simulink library "SUB_ECU_L4_MABX_HW_Interface_PIC_KW"  (R2018a)
settings: Solver=VariableStepAuto  StartTime=0.0  StopTime=10.0  RelTol=1e-3
PostLoadFcn:
  | , if any(exist('dsrtsu_mdlpostloadfcn', 'file') == [2, 3, 6]), try dsrtsu_mdlpostloadfcn('Execute', bdroot); catch fprintf('Error in PostLoadFcn (dsrtsu_mdlpostloadfcn) for model "%s":\n %s\n', bdroot, lasterr); end, end,
undefined symbols (not defined in the file or in its folder): CANR_PROPB_REAX_3_13_CHANNEL_APV, CANR_PROPB_REAX_4_13_CHANNEL_APV, CANR_PROPB_XPR_1_50_CHANNEL_APV, ENUM_CAN_RX_T, ENUM_CAN_TX_T, ENUM_REAX_OPERATION_MODE_T, ENUM_SIGNAL_HEALTH_T, ENUM_XBR_CONTROL_MODE_T, ENUM_XBR_EBI_MODE_T, ENUM_XBR_PASS_THROUGH_ACTIVE_T, ENUM_XBR_PRIORITY_T, ENUM_XPR_INHIBIT_PARK_MANUAL_T, ENUM_XPR_INHIBIT_UNPARK_MANUAL_T, ENUM_XPR_PARK_MANUAL_T, ENUM_XPR_UNPARK_MANUAL_T, PROPB_REAX_1_E4_DES_POS_SIG_SRC_APV, PROPB_REAX_1_E4_DESIRED_OPMODE_APV, PROPB_REAX_1_E4_DESIRED_POSITION_APV, PROPB_REAX_CHANNEL_APV, ptc_matlab_lib
libraries: PTC_MBDS_LIB x292, rtican x158, simulink x58, EmE_MBD_Blockset x38, rti1401lib_dio_type4 x13, simulink_need_slupdate x7, rti1401lib_adc_type4 x3, rtmapslib x3, $bdroot x3, dsa_tcpip_lib x2, SUB_ECU_L4_MABX_HW_Interface_PTC_1571 x1, rtitasklib x1
(part 7 of 48)

== system SUB_ECU_L4_MABX_HW_Interface_PIC_KW/CAN_Out_PIC_KW/CAN_TX_20ms/Encode_PropB_XBR_B3 ==
  note: This might cause a limit cycle, why switch pass through mode based on braking error
  In : Inport
  Bus Creator1 : BusCreator  Inputs=7
  Bus Creator2 : BusCreator  Inputs=7
  Bus Selector2 : BusSelector  OutputSignals=10msTask.BrakeCtrl.BrakingPID_Y,10msTask.BrakeCtrl.BrakingControlActive,INPUTS.DIO_Bus.OperatorEnableSwitch
  Constant10 : Constant  Value=ENUM_XBR_PASS_THROUGH_ACTIVE_T.NOT_ACTIVE
  Constant2 : Constant  Value=-15.687
  Constant4 : Constant  Value=0
  Constant7 : Constant  Value=ENUM_XBR_PASS_THROUGH_ACTIVE_T.ACTIVE
  Constant8 : Constant  Value=ENUM_XBR_PASS_THROUGH_ACTIVE_T.ERROR
  Constant9 : Constant  Value=ENUM_XBR_PASS_THROUGH_ACTIVE_T.NOT_AVAILABLE
  DECEL_GOV_XBR_URGENCY_MPV : Lookup_n-D  NumberOfTableDimensions=1  BreakpointsForDimension1=[-15.687 -2 -1.5 -1.2 -1.1 -1 -0.9 0]  Table=[100 50 20 15 15 15 10 10]  ExtrapMethod=Clip  UseLastTableValue=on  InputSameDT=on
      settings: AttributesFormatString=|
      | X: %<BreakpointsForDimension1>
      | Y: %<Table>
  Divide1 : Product  Inputs=**  InputSameDT=on
  If_Then_Else : EmE_MBD_Blockset/Signal Routing/If_Then_Else
      settings: SourceProductName=PACCAR EmE MBD Blockset
  Multiport Switch : MultiPortSwitch  DataPortOrder=Zero-based contiguous  Inputs=4  DiagnosticForDefault=None  zeroidx=on  InputSameDT=on
  Switch1 : Switch  Criteria=u2 ~= 0
  Terminator1 : Terminator
  XBRControlMode : Constant  Value=ENUM_XBR_CONTROL_MODE_T.ACCEL_CTRL_WITH_MAX_MODE
  XBRControlModeOVR : Constant  Value=ENUM_XBR_CONTROL_MODE_T.ACCEL_CTRL_WITH_MAX_MODE
  XBREnduranceBrakeIntegrationMode : Constant  Value=ENUM_XBR_EBI_MODE_T.EBI_ALLOWED
  XBREnduranceBrakeIntegrationModeOVR : Constant  Value=ENUM_XBR_EBI_MODE_T.EBI_ALLOWED
  XBRExternalAccelDemandOVR : Constant  Value=0
  XBRPassThroughActiveOVR : Constant  Value=ENUM_XBR_PASS_THROUGH_ACTIVE_T.ACTIVE
  XBRPassThroughEnabled : Constant
  XBRPassThroughEnabledOVR : Constant
  XBRPriority : Constant  Value=ENUM_XBR_PRIORITY_T.MEDIUM_PRIORITY
  XBRPriorityOVR : Constant  Value=ENUM_XBR_PRIORITY_T.MEDIUM_PRIORITY
  XBRUrgency : Constant  Value=25
  XBRUrgencyOVR : Constant  Value=25
  XBRValueOverride : Constant  Value=false
  Out : Outport
  wires:
  Constant4/1 -> Switch1/3
  Divide1/1 -> Switch1/1  "XBRExternalAccelDemand"
  Bus Selector2/3 -> Switch1/2  "<OperatorEnableSwitch>"
  Multiport Switch/1 -> Bus Creator1/5  "XBRPassThroughActive"
  DECEL_GOV_XBR_URGENCY_MPV/1 -> Terminator1/1  "XBRUrgency"
  Constant10/1 -> Multiport Switch/2
  Switch1/1 -> Bus Creator1/1, DECEL_GOV_XBR_URGENCY_MPV/1  "XBRExternalAccelDemand"
  Constant2/1 -> Divide1/2
  In/1 -> Bus Selector2/1
  Constant8/1 -> Multiport Switch/4
  Constant9/1 -> Multiport Switch/5
  Constant7/1 -> Multiport Switch/3
  XBREnduranceBrakeIntegrationMode/1 -> Bus Creator1/2  "XBREnduranceBrakeIntegrationMode"
  Bus Selector2/1 -> Divide1/1  "<BrakingPID_Y>"
  Bus Creator1/1 -> If_Then_Else/3
  XBRUrgency/1 -> Bus Creator1/6  "XBRUrgency"
  Bus Selector2/2 -> Multiport Switch/1  "<BrakingControlActive>"
  XBRControlMode/1 -> Bus Creator1/4  "XBRControlMode"
  XBRPriority/1 -> Bus Creator1/3  "XBRPriority"
  XBRPassThroughEnabled/1 -> Bus Creator1/7  "XBRPassThroughEnabled"
  XBRValueOverride/1 -> If_Then_Else/1
  If_Then_Else/1 -> Out/1
  XBRPassThroughActiveOVR/1 -> Bus Creator2/5  "XBRPassThroughActive"
  XBREnduranceBrakeIntegrationModeOVR/1 -> Bus Creator2/2  "XBREnduranceBrakeIntegrationMode"
  XBRExternalAccelDemandOVR/1 -> Bus Creator2/1  "XBRExternalAccelDemand"
  XBRUrgencyOVR/1 -> Bus Creator2/6  "XBRUrgency"
  XBRControlModeOVR/1 -> Bus Creator2/4  "XBRControlMode"
  XBRPriorityOVR/1 -> Bus Creator2/3  "XBRPriority"
  XBRPassThroughEnabledOVR/1 -> Bus Creator2/7  "XBRPassThroughEnabled"
  Bus Creator2/1 -> If_Then_Else/2

== system SUB_ECU_L4_MABX_HW_Interface_PIC_KW/CAN_Out_PIC_KW/CAN_TX_5000ms/CAN_TX_RQST_13_E4 ==
  RawData : Inport
  OperatorEnable : Inport  Port=2
  Data Type Conversion6 : DataTypeConversion  OutDataTypeStr=boolean  SaturateOnIntegerOverflow=on
  Enable_TX_RequestDiagMsgFromREAX : Constant  Value=boolean(1)
  TX_CAN5 : Subsystem
  wires:
  OperatorEnable/1 -> TX_CAN5/3(OperatorEnable)
  Enable_TX_RequestDiagMsgFromREAX/1 -> Data Type Conversion6/1
  Data Type Conversion6/1 -> TX_CAN5/1(Enable)
  RawData/1 -> TX_CAN5/2(RawData)

== system SUB_ECU_L4_MABX_HW_Interface_PIC_KW/CAN_Out_PIC_KW/CAN_TX_5000ms/Encode_RQST ==
  PGN : Inport
  AND : PTC_MBDS_LIB/MBDS Standard Library/Basic Operations/Logic and Bit Operations/AND  BitwiseMode=on  Inputs=1  UseBitMask=on  BitMask='000000FF'  OutDataTypeStr=uint8  PTC_MBDS_BlockVersion=5.41  PTC_BlockType=PTC_MBDS_AND
      settings: AttributesFormatString=bitwise  SourceProductName=PACCAR Technical Center MBDS Library
  AND1 : PTC_MBDS_LIB/MBDS Standard Library/Basic Operations/Logic and Bit Operations/AND  BitwiseMode=on  Inputs=1  UseBitMask=on  BitMask='0000FF00'  OutDataTypeStr=uint16  PTC_MBDS_BlockVersion=5.41  PTC_BlockType=PTC_MBDS_AND
      settings: AttributesFormatString=bitwise  SourceProductName=PACCAR Technical Center MBDS Library
  AND2 : PTC_MBDS_LIB/MBDS Standard Library/Basic Operations/Logic and Bit Operations/AND  BitwiseMode=on  Inputs=1  UseBitMask=on  BitMask='00FF0000'  OutDataTypeStr=uint32  PTC_MBDS_BlockVersion=5.41  PTC_BlockType=PTC_MBDS_AND
      settings: AttributesFormatString=bitwise  SourceProductName=PACCAR Technical Center MBDS Library
  Data Type Conversion : DataTypeConversion  OutDataTypeStr=uint32  SaturateOnIntegerOverflow=on
  Data Type Conversion1 : DataTypeConversion  OutDataTypeStr=uint8  SaturateOnIntegerOverflow=on
  Data Type Conversion2 : DataTypeConversion  OutDataTypeStr=uint8  SaturateOnIntegerOverflow=on
  Data Type Conversion3 : DataTypeConversion  OutDataTypeStr=uint8  SaturateOnIntegerOverflow=on
  Mux : Mux  Inputs=3
  "Shift_Arithmetic " : ArithShift  BitShiftNumber=8
  Shift_Arithmetic 1 : ArithShift  BitShiftNumber=16
  Data : Outport
  wires:
  Data Type Conversion3/1 -> Mux/1
  Mux/1 -> Data/1
  Data Type Conversion2/1 -> Mux/3
  Data Type Conversion1/1 -> Mux/2
  Shift_Arithmetic 1/1 -> Data Type Conversion2/1
  AND2/1 -> Shift_Arithmetic 1/1
  "Shift_Arithmetic "/1 -> Data Type Conversion1/1
  AND1/1 -> "Shift_Arithmetic "/1
  AND/1 -> Data Type Conversion3/1
  Data Type Conversion/1 -> AND/1, AND1/1, AND2/1
  PGN/1 -> Data Type Conversion/1

== system SUB_ECU_L4_MABX_HW_Interface_PIC_KW/CAN_Out_PIC_KW/CAN_TX_5000ms/RQST_13_E4_PGN ==
  Repeating_Sequence_Stair : PTC_MBDS_LIB/Extras/Sources/Repeating_Sequence_Stair  OutValues=uint32([65527, 65226, 65227, 65235, 65242, 65259, 65267, 65260])  OutValues_prev=uint32([65527, 65226, 65227, 65235, 65242, 65259, 65267, 65260])  PTC_MBDS_BlockVersion=5.41  PTC_BlockType=PTC_MBDS_Repeating_Sequence_Stair
      settings: SourceProductName=PACCAR Technical Center MBDS Library
  PGN : Outport
  wires:
  Repeating_Sequence_Stair/1 -> PGN/1

== system SUB_ECU_L4_MABX_HW_Interface_PIC_KW/CAN_Out_PIC_KW/CAN_TX_50ms/CAN_TX_CCVS1 ==
  In1 : Inport
  enable : Inport  Port=2
  Bus Selector : BusSelector  OutputSignals=INPUTS.CAN.CCVS1_00.CCVS1Data.TwoSpeedAxleSwitch,INPUTS.CAN.CCVS1_00.CCVS1Data.ParkingBrakeSwitch,INPUTS.CAN.CCVS1_00.CCVS1Data.CruiseCtrlPauseSwitch,INPUTS.CAN.CCVS1_00.CCVS1Data.ParkBrakeReleaseInhibitRq,INPUTS.CAN.CCVS1_00.CCVS1Data.WheelBasedVehicleSpeed,INPUTS.CAN.CCVS1_00.CCVS1Data.CruiseCtrlActive,INPUTS.CAN.CCVS1_00.CCVS1Data.CruiseCtrlEnableSwitch,INPUTS.CAN.CCVS1_00.CCVS1Data.BrakeSwitch,INPUTS.CAN.CCVS1_00.CCVS1Data.ClutchSwitch,INPUTS.CAN.CCVS1_00.CCVS1Data.CruiseCtrlSetSwitch,INPUTS.CAN.CCVS1_00.CCVS1Data.CruiseCtrlCoastSwitch,INPUTS.CAN.CCVS1_00.CCVS1Data.CruiseCtrlResumeSwitch,INPUTS.CAN.CCVS1_00.CCVS1Data.CruiseCtrlAccelerateSwitch,INPUTS.CAN.CCVS1_00.CCVS1Data.CruiseCtrlSetSpeed,INPUTS.CAN.CCVS1_00.CCVS1Data.PTOGovernorState,INPUTS.CAN.CCVS1_00.CCVS1Data.CruiseCtrlStates,INPUTS.CAN.CCVS1_00.CCVS1Data.EngIdleIncrementSwitch,INPUTS.CAN.CCVS1_00.CCVS1Data.EngIdleDecrementSwitch,INPUTS.CAN.CCVS1_00.CCVS1Data.EngTestModeSwitch,INPUTS.CAN.CCVS1_00.CCVS1Data.EngShutdownOverrideSwitch
  CCVS1_E3 : rtican/RTICAN Transmit (TX)   Reserved1=[]  Reserved2=[]  Reserved3=[]  Reserved4=[]  SfcnMessage=[]  Msg_Struct=[]  BoardTypeNo=[]  BoardNo=[]  ChannelNo=[]  Parameters=[]  DialogFcn=[]  UnitName=[]  Revision=[]  UnitValues=[]  DSProperties=struct('RTI',struct('Version',uint32(5),'BlockType',struct('isSLSource',uint8(1),'isSLSink',uint8(1),'isHWSource',uint8(0),'isHWSink',uint8(0),'isSetup',uint8(0),'isInline',uint8(1),'isNonInline',uint8(0),'isInterrupt',uint8(0),'isChannelwise',uint8(0)),'IOBoardType','RTICAN','UnitType','MESSAGE','Identifier','TX','DialogType','MSVC','BlockSet','RTICAN','SlaveProcessor','CAN'))  RTIBlockInterface=struct('InputPortsWidth',int32([1 1 1 1 1 1 1 1 1 1 1 1 1 1 1 1 1 1 1 1]),'InputPortsActive',ones(1,20),'InputPortsName',{{'SPN69_TwoSpeedAxleSwitch','SPN70_ParkingBrakeSwitch','SPN1633_CruiseControlPauseSwitch','SPN3807_ParkBrakeReleaseInhReq','SPN84_WheelBasedVehicleSpeed','SPN595_CruiseControlActive','SPN596_CruiseControlEnableSwitch','SPN597_BrakeSwitch','SPN598_ClutchSwitch','SPN599_CruiseControlSetSwitch','SPN600_CruiseControlCoastDecelSw','SPN601_CruiseControlResumeSwitch','SPN602_CruiseControlAccelerateSw','SPN86_CruiseControlSetSpeed','SPN976_PTOGovernorState','SPN527_CruiseControlStates','SPN968_EngIdleIncrementSw','SPN967_EngIdleDecrementSwitch','SPN966_EngDiagTestModeSwitch','SPN1237_EngShutdownOvrdSwitch'}},'InputPortsDataType',{{'SS_DOUBLE','SS_DOUBLE','SS_DOUBLE','SS_DOUBLE','SS_DOUBLE','SS_DOUBLE','SS_DOUBLE','SS_DOUBLE','SS_DOUBLE','SS_DOUBLE','SS_DOUBLE','SS_DOUBLE','SS_DOUBLE','SS_DOUBLE','SS_DOUBLE','SS_DOUBLE','SS_DOUBLE','SS_DOUBLE','SS_DOUBLE','SS_DOUBLE'}},'OutputPortsWidth',int32([1 1 1 1]),'OutputPortsActive',[1 1 1 1],'OutputPortsName',{{['TX status'],['TX time'],['TX delta time'],['TX delay time']}},'DialogFcn','rtican_message_interface_gui','BlockDisplay',{{'','center'}},'IconTransparency','on','InitLevel',3,'BlockName',struct('Token',{{'CCVS1_E3'}}),'SampleTime',{{-1}},'TriggerPort',{{'none'}},'EnablePort',{{'yes'}})  RTIBlockParameters="struct('BoardTypeNo',{{1,'OFF',[]}},'BoardNo',{{2,'ON',[1 16]}},'ChannelNo',{{1,'ON',[1 2]}},'Parameters',{{struct('DataFileSupport',struct('DataFileSelectedMaster',1,'DataFileSelectedLocal',0,'DataFileName',['c:\\users\\gavin.coelho\\repos\\l4 svn\\branches\\gennaro\\project_l4\\src\\projectlibrary\\dbc\\mabx_can1.dbc|'],'DataFileDate',{{{['10-Feb-2017 15:17:27']}}},'SelectedFile',['<no file selected>']),'Options',struct('StatusSelected',1,'TimeSelected',1,'DeltaTimeSelected',1,'DelayTimeSelected',1,'DelayTimeTXCommandSelected',0,'EncodeSetUnusedBitsToOne',0,'EnableMsgLoopback',0,'TriggerPort',struct('Selected',0,'TriggerType',0),'EnablePortSelected',1,'SignalOnPortnameSelected',1,'UserCoding',struct('Selected',0,'InterfaceFile','UserEncodingFile','FcnName','UserEncodeFcn','InportSelected',0,'InportWidth',1,'OutportSelected',0,'OutportWidth',1),'TerminationMsg',struct('Selected',0,'Byte0_7','0'),'InitialMsg',struct('Selected',0,'Byte0_7','0')),'Message',struct('MsgOnBlocknameSelected',1,'MsgName','CCVS1_E3','MsgIdFormat',1,'MsgId',419361251,'MsgLength',8,'NumSignals',20,'SampleTime',-1,'StartTime',struct('Selected',0,'Value',0),'AutoRepeatTime',struct('Selected',0,'Value',0.1),'Timeout',struct('Selected',0,'Value',0.1),'DelayTime',struct('Selected',0,'Value',0.1),'Signal',struct('SgnName',{'SPN69_TwoSpeedAxleSwitch','SPN70_ParkingBrakeSwitch','SPN1633_CruiseControlPauseSwitch','SPN3807_ParkBrakeReleaseInhReq','SPN84_WheelBasedVehicleSpeed','SPN595_CruiseControlActive','SPN596_CruiseControlEnableSwitch','SPN597_BrakeSwitch','SPN598_ClutchSwitch','SPN599_CruiseControlSetSwitch','SPN600_CruiseControlCoastDecelSw','SPN601_CruiseControlResumeSwitch','SPN602_CruiseControlAccelerateSw','SPN86_CruiseControlSetSpeed','SPN976_PTOGovernorState','SPN527_CruiseControlStates','SPN968_EngIdleIncrementSw','SPN967_EngIdleDecrementSwitch','SPN966_EngDiagTestModeSwitch','SPN1237_EngShutdownOvrdSwitch'},'SgnStartBit',{0,2,4,6,8,24,26,28,30,32,34,36,38,40,48,53,56,58,60,62},'SgnLength',{2,2,2,2,16,2,2,2,2,2,2,2,2,8,5,3,2,2,2,2},'SgnType',{0,0,0,0,0,0,0,0,0,0,0,0,0,0,0,0,0,0,0,0},'ModeValue',{-1,-1,-1,-1,-1,-1,-1,-1,-1,-1,-1,-1,-1,-1,-1,-1,-1,-1,-1,-1},'DataType',{0,0,0,0,0,0,0,0,0,0,0,0,0,0,0,0,0,0,0,0},'ByteLayout',{0,0,0,0,0,0,0,0,0,0,0,0,0,0,0,0,0,0,0,0},'Factor',{1,1,1,1,2^-8,1,1,1,1,1,1,1,1,1,1,1,1,1,1,1},'Offset',{0,0,0,0,0,0,0,0,0,0,0,0,0,0,0,0,0,0,0,0},'SgnComment',{{['Switch signal which indicates the current axle range.']},{['Switch signal which indicates when the parking brake is set.']},{['Switch signal which indicates the position of the Cruise Control Pause Switch used on Remote Cruise Control applications. The Cruise Control Pause Switch signal temporarily disables the Cruise Control function']},{['Park Brake Release Inhibit Request signals the desire that an applied park brake remain applied and limit the ability of the vehicle to be moved']},{['Speed of the vehicle as calculated from wheel or tailshaft speed.']},{['Cruise control is switched on or off']},{['Switch signal which indicates that it is possible to manage the cruise control function.']},{['Switch signal which indicates that the driver operated brake foot pedal is being pressed.']},{['Switch signal which indicates that the clutch pedal is being pressed.']},{['Switch signal of the cruise control activator which indicates that the activator is in the position “set.”']},{['Switch signal of the cruise control activator which indicates that the activator is in the position “coast (decelerate).”']},{['Switch signal of the cruise control activator which indicates that the activator is in the position “resume.”']},{['Switch signal of the cruise control activator which indicates that the activator is in the position “accelerate.”']},{['Value of set (chosen) velocity of velocity control system.  See SPN 6809 for an alternate resolution.']},{['This parameter is used to indicate the current state or mode of operation by the power takeoff (PTO) governor.']},{['This parameter is used to indicate the current state, or mode, of operation by the cruise control device.  This is a status parameter.']},{['Switch signal which indicates the position of the idle increment switch.']},{['Switch signal which indicates the position of the idle decrement switch.']},{['Switch signal which indicates the position of the engine diagnostic test mode switch.']},{['Switch signal which indicates the position of the engine shutdown override switch.  This switch function allows the operator to override an impending engine shutdown.']}},'SgnUnit',{'','','','','km/h','','','','','','','','','km/h','','','','','',''},'Min',{0,0,0,0,0,0,0,0,0,0,0,0,0,0,0,0,0,0,0,0},'Max',{0,0,0,0,0,0,0,0,0,0,0,0,0,0,0,0,0,0,0,0},'SLDataType',{'SS_DOUBLE','SS_DOUBLE','SS_DOUBLE','SS_DOUBLE','SS_DOUBLE','SS_DOUBLE','SS_DOUBLE','SS_DOUBLE','SS_DOUBLE','SS_DOUBLE','SS_DOUBLE','SS_DOUBLE','SS_DOUBLE','SS_DOUBLE','SS_DOUBLE','SS_DOUBLE','SS_DOUBLE','SS_DOUBLE','SS_DOUBLE','SS_DOUBLE'}),'MsgIdNumFormat',1,'MsgComment',{{['Cruise Control/Vehicle Speed 1 (Special CECU source address: 0xE3)']}}),'Version',1.2,'general',struct('isFromLib',0)),'OFF',[]}},'GroupId',{{struct('Group',{{'RTICAN'}},'No',3,'Behavior',{{'NAMECHANGE'}},'BlockType',{{'SINK'}},'NameChangeFlag',0),'OFF',[]}},'SFcnRTICANMessage',{{struct('MsgType','TX','SFcnPortType','Scalar','MsgName','CCVS1_E3','MsgIdFormat','XTD','MsgId',419361251,'MsgLength',8,'NumSignals',20,'SampleTime',-1,'StartTime',struct('Selected','no','Value',0),'AutoRepeatTime',struct('Selected','no','Value',0.1),'Timeout',struct('Selected','no','Value',0.1),'Signal',struct('SgnName',{'SPN69_TwoSpeedAxleSwitch','SPN70_ParkingBrakeSwitch','SPN1633_CruiseControlPauseSwitch','SPN3807_ParkBrakeReleaseInhReq','SPN84_WheelBasedVehicleSpeed','SPN595_CruiseControlActive','SPN596_CruiseControlEnableSwitch','SPN597_BrakeSwitch','SPN598_ClutchSwitch','SPN599_CruiseControlSetSwitch','SPN600_CruiseControlCoastDecelSw','SPN601_CruiseControlResumeSwitch','SPN602_CruiseControlAccelerateSw','SPN86_CruiseControlSetSpeed','SPN976_PTOGovernorState','SPN527_CruiseControlStates','SPN968_EngIdleIncrementSw','SPN967_EngIdleDecrementSwitch','SPN966_EngDiagTestModeSwitch','SPN1237_EngShutdownOvrdSwitch'},'SgnStartBit',{0,2,4,6,8,24,26,28,30,32,34,36,38,40,48,53,56,58,60,62},'SgnLength',{2,2,2,2,16,2,2,2,2,2,2,2,2,8,5,3,2,2,2,2},'SgnType',{'standard','standard','standard','standard','standard','standard','standard','standard','standard','standard','standard','standard','standard','standard','standard','standard','standard','standard','standard','standard'},'ModeValue',{-1,-1,-1,-1,-1,-1,-1,-1,-1,-1,-1,-1,-1,-1,-1,-1,-1,-1,-1,-1},'DataType',{['unsigned int'],['unsigned int'],['unsigned int'],['unsigned int'],['unsigned int'],['unsigned int'],['unsigned int'],['unsigned int'],['unsigned int'],['unsigned int'],['unsigned int'],['unsigned int'],['unsigned int'],['unsigned int'],['unsigned int'],['unsigned int'],['unsigned int'],['unsigned int'],['unsigned int'],['unsigned int']},'ByteLayout',{['little endian'],['little endian'],['little endian'],['little endian'],['little endian'],['little endian'],['little endian'],['little endian'],['little endian'],['little endian'],['little endian'],['little endian'],['little endian'],['little endian'],['little endian'],['little endian'],['little endian'],['little endian'],['little endian'],['little endian']},'Factor',{1,1,1,1,2^-8,1,1,1,1,1,1,1,1,1,1,1,1,1,1,1},'Offset',{0,0,0,0,0,0,0,0,0,0,0,0,0,0,0,0,0,0,0,0},'SLDataType',{'SS_DOUBLE','SS_DOUBLE','SS_DOUBLE','SS_DOUBLE','SS_DOUBLE','SS_DOUBLE','SS_DOUBLE','SS_DOUBLE','SS_DOUBLE','SS_DOUBLE','SS_DOUBLE','SS_DOUBLE','SS_DOUBLE','SS_DOUBLE','SS_DOUBLE','SS_DOUBLE','SS_DOUBLE','SS_DOUBLE','SS_DOUBLE','SS_DOUBLE'}),'StatusSelected','yes','TimeSelected','yes','DeltaTimeSelected','yes','DelayTimeSelected','yes','DelayTimeTXCommandSelected','no','EncodeSetUnusedBitsToOne','no','EnableMsgLoopback','no','TriggerPort',struct('Selected','no','TriggerType',0),'EnablePortSelected','yes','UserCoding',struct('Selected','no','InterfaceFile','UserEncodingFile','FcnName','UserEncodeFcn','InportSelected','no','InportWidth',1,'OutportSelected','no','OutportWidth',1),'TerminationMsg',struct('Selected','no','Byte0','0x00','Byte1','0x00','Byte2','0x00','Byte3','0x00','Byte4','0x00','Byte5','0x00','Byte6','0x00','Byte7','0x00'),'InitialMsg',struct('Selected','no','Byte0','0x00','Byte1','0x00','Byte2','0x00','Byte3','0x00','Byte4','0x00','Byte5','0x00','Byte6','0x00','Byte7','0x00'),'BoardType','DS1','BoardNo',2,'ControllerNo',1),'OFF',[]}},'TLCFileName',{{'rtican_tx_message','OFF',[]}})"  RTISFcnParameters=struct('SFcnRTICANMessage','struct','TLCFileName','char')  RTIBlockParaDefault=struct('BoardTypeNo',4302,'BoardNo',1,'ChannelNo',1,'Parameters',struct('DataFileSupport',struct('DataFileSelectedMaster',0,'DataFileSelectedLocal',0,'DataFileName','','DataFileDate','','SelectedFile',['<no file selected>']),'Options',struct('StatusSelected',1,'TimeSelected',1,'DeltaTimeSelected',1,'DelayTimeSelected',1,'DelayTimeTXCommandSelected',0,'EncodeSetUnusedBitsToOne',0,'EnableMsgLoopback',0,'TriggerPort',struct('Selected',0,'TriggerType','rising'),'EnablePortSelected',0,'SignalOnPortnameSelected',1,'UserCoding',struct('Selected',0,'InterfaceFile','UserEncodingFile','FcnName','UserEncodeFcn','InportSelected',0,'InportWidth',1,'OutportSelected',0,'OutportWidth',1),'TerminationMsg',struct('Selected',0,'Byte0_7','0'),'InitialMsg',struct('Selected',0,'Byte0_7','0')),'Message',struct('MsgOnBlocknameSelected',0,'MsgName',['TX Message'],'MsgIdFormat',0,'MsgId',100,'MsgLength',8,'NumSignals',1,'SampleTime',-1,'StartTime',struct('Selected',0,'Value',0),'AutoRepeatTime',struct('Selected',0,'Value',0.1),'Timeout',struct('Selected',0,'Value',0.1),'DelayTime',struct('Selected',0,'Value',0.1),'Signal',struct('SgnName',['TX signal'],'SgnStartBit',0,'SgnLength',8,'SgnType',0,'ModeValue',-1,'DataType',0,'SLDataType','SS_DOUBLE','ByteLayout',0,'Factor',1,'Offset',0,'Min',0,'Max',255,'SgnComment',{{}},'SgnUnit',''),'MsgIdNumFormat',0,'MsgComment',{{''}}),'Version',1.2,'general',struct('isFromLib',1)),'GroupId',struct('Group',{{'RTICAN'}},'No',1,'Behavior',{{'NAMECHANGE'}},'BlockType',{{'SINK'}},'NameChangeFlag',0),'SFcnRTICANMessage',struct('MsgType','TX','MsgName',['TX Message'],'MsgIdFormat','STD','MsgId',100,'MsgLength',2,'NumSignals',1,'SampleTime',-1,'StartTime',struct('Selected','no','Value',0),'AutoRepeatTime',struct('Selected','no','Value',0.1),'Timeout',struct('Selected','no','Value',0.1),'DelayTime',struct('Selected','no','Value',0.1),'Signal',struct('SgnName',['TX signal'],'SgnStartBit',0,'SgnLength',8,'SgnType','standard','ModeValue',-1,'DataType',['unsigned int'],'ByteLayout',['little endian'],'SLDataType','SS_DOUBLE','Factor',1,'Offset',0),'StatusSelected','yes','TimeSelected','yes','DeltaTimeSelected','yes','DelayTimeSelected','yes','EnablePortSelected','no','EnableMsgLoopback','no','DelayTimeTXCommandSelected','no','EncodeSetUnusedBitsToOne','no','UserCoding',struct('Selected','no','InterfaceFile','UserDecodingFile','FcnName','UserDecodeFcn','InportSelected','no','InportWidth',1,'OutportSelected','no','OutportWidth',1),'TerminationMsg',struct('Selected','no','Byte0','0x00','Byte1','0x00','Byte2','0x00','Byte3','0x00','Byte4','0x00','Byte5','0x00','Byte6','0x00','Byte7','0x00'),'InitialMsg',struct('Selected','no','Byte0','0x00','Byte1','0x00','Byte2','0x00','Byte3','0x00','Byte4','0x00','Byte5','0x00','Byte6','0x00','Byte7','0x00'),'TriggerPort',struct('Selected','no','TriggerType','rising'),'BoardType','DS4302','BoardNo',1,'ControllerNo',1,'SFcnPortType','Scalar'),'TLCFileName','rtican_tx_message')
      settings: AttributesFormatString=Group Id: RTICAN3\n  SourceProductName=dSPACE RTI CAN Blockset
  Terminator{,1..3} (4 alike) : Terminator
  wires:
  enable/1 -> CCVS1_E3/Enable
  Bus Selector/20 -> CCVS1_E3/20  "<EngShutdownOverrideSwitch>"
  Bus Selector/19 -> CCVS1_E3/19  "<EngTestModeSwitch>"
  Bus Selector/18 -> CCVS1_E3/18  "<EngIdleDecrementSwitch>"
  Bus Selector/17 -> CCVS1_E3/17  "<EngIdleIncrementSwitch>"
  Bus Selector/16 -> CCVS1_E3/16  "<CruiseCtrlStates>"
  Bus Selector/15 -> CCVS1_E3/15  "<PTOGovernorState>"
  Bus Selector/14 -> CCVS1_E3/14  "<CruiseCtrlSetSpeed>"
  Bus Selector/13 -> CCVS1_E3/13  "<CruiseCtrlAccelerateSwitch>"
  Bus Selector/12 -> CCVS1_E3/12  "<CruiseCtrlResumeSwitch>"
  Bus Selector/11 -> CCVS1_E3/11  "<CruiseCtrlCoastSwitch>"
  Bus Selector/10 -> CCVS1_E3/10  "<CruiseCtrlSetSwitch>"
  Bus Selector/9 -> CCVS1_E3/9  "<ClutchSwitch>"
  Bus Selector/8 -> CCVS1_E3/8  "<BrakeSwitch>"
  Bus Selector/7 -> CCVS1_E3/7  "<CruiseCtrlEnableSwitch>"
  Bus Selector/6 -> CCVS1_E3/6  "<CruiseCtrlActive>"
  Bus Selector/5 -> CCVS1_E3/5  "<WheelBasedVehicleSpeed>"
  Bus Selector/4 -> CCVS1_E3/4  "<ParkBrakeReleaseInhibitRq>"
  Bus Selector/3 -> CCVS1_E3/3  "<CruiseCtrlPauseSwitch>"
  Bus Selector/2 -> CCVS1_E3/2  "<ParkingBrakeSwitch>"
  Bus Selector/1 -> CCVS1_E3/1  "<TwoSpeedAxleSwitch>"
  CCVS1_E3/1 -> Terminator/1
  CCVS1_E3/2 -> Terminator1/1
  CCVS1_E3/3 -> Terminator2/1
  CCVS1_E3/4 -> Terminator3/1
  In1/1 -> Bus Selector/1

== system SUB_ECU_L4_MABX_HW_Interface_PIC_KW/CAN_Out_PIC_KW/CAN_TX_50ms/CAN_TX_TC1_05 ==
  In1 : Inport
  Bus Selector : BusSelector  OutputSignals=INPUTS.CAN.TC1_05.SPN681_TransGearShiftInhibitReq,INPUTS.CAN.TC1_05.SPN682_TransTrqConvLockupDisReq,INPUTS.CAN.TC1_05.SPN683_DisengageDrivelineReq,INPUTS.CAN.TC1_05.SPN4242_TransRevGearShiftInhibRq,INPUTS.CAN.TC1_05.SPN684_RequestedPercClutchSlip,INPUTS.CAN.TC1_05.SPN525_TransRequestedGear,INPUTS.CAN.TC1_05.SPN685_DisengageDiffLockRqFrAx1,INPUTS.CAN.TC1_05.SPN686_DisengageDiffLockRqFrAx2,INPUTS.CAN.TC1_05.SPN687_DisengageDiffLockRqRrAx1,INPUTS.CAN.TC1_05.SPN688_DisengageDiffLockRqRrAx2,INPUTS.CAN.TC1_05.SPN689_DisengageDiffLockRqC,INPUTS.CAN.TC1_05.SPN690_DisengageDiffLockRqCF,INPUTS.CAN.TC1_05.SPN691_DisengageDiffLockRqCR,INPUTS.CAN.TC1_05.SPN5762_TransLoadRedInhibitRq,INPUTS.CAN.TC1_05.SPN1852_TransmissionMode1,INPUTS.CAN.TC1_05.SPN1853_TransmissionMode2,INPUTS.CAN.TC1_05.SPN1854_TransmissionMode3,INPUTS.CAN.TC1_05.SPN1855_TransmissionMode4,INPUTS.CAN.TC1_05.SPN7695_TransAutoNeutralRequest,INPUTS.CAN.TC1_05.SPN4255_TransRequestedLaunchGear,INPUTS.CAN.TC1_05.SPN2985_TransShiftSelDispModeSw,INPUTS.CAN.TC1_05.SPN4246_TransmissionMode5,INPUTS.CAN.TC1_05.SPN4247_TransmissionMode6,INPUTS.CAN.TC1_05.SPN4248_TransmissionMode7,INPUTS.CAN.TC1_05.SPN4249_TransmissionMode8,INPUTS.CAN.TC1_05.RX_status
  CANT_TC1_03_05_APV : Constant  Value=false
  TC1_03_05 : rtican/RTICAN Transmit (TX)   Reserved1=[]  Reserved2=[]  Reserved3=[]  Reserved4=[]  SfcnMessage=[]  Msg_Struct=[]  BoardTypeNo=[]  BoardNo=[]  ChannelNo=[]  Parameters=[]  DialogFcn=[]  UnitName=[]  Revision=[]  UnitValues=[]  DSProperties=struct('RTI',struct('Version',uint32(5),'BlockType',struct('isSLSource',uint8(1),'isSLSink',uint8(1),'isHWSource',uint8(0),'isHWSink',uint8(0),'isSetup',uint8(0),'isInline',uint8(1),'isNonInline',uint8(0),'isInterrupt',uint8(0),'isChannelwise',uint8(0)),'IOBoardType','RTICAN','UnitType','MESSAGE','Identifier','TX','DialogType','MSVC','BlockSet','RTICAN','SlaveProcessor','CAN'))  RTIBlockInterface=struct('InputPortsWidth',int32([1 1 1 1 1 1 1 1 1 1 1 1 1 1 1 1 1 1 1 1 1 1 1 1 1]),'InputPortsActive',ones(1,25),'InputPortsName',{{'SPN681_TransGearShiftInhibitReq','SPN682_TransTrqConvLockupDisReq','SPN683_DisengageDrivelineReq','SPN4242_TransRevGearShiftInhibRq','SPN684_RequestedPercClutchSlip','SPN525_TransRequestedGear','SPN685_DisengageDiffLockRqFrAx1','SPN686_DisengageDiffLockRqFrAx2','SPN687_DisengageDiffLockRqRrAx1','SPN688_DisengageDiffLockRqRrAx2','SPN689_DisengageDiffLockRqC','SPN690_DisengageDiffLockRqCF','SPN691_DisengageDiffLockRqCR','SPN5762_TransLoadRedInhibitRq','SPN1852_TransmissionMode1','SPN1853_TransmissionMode2','SPN1854_TransmissionMode3','SPN1855_TransmissionMode4','SPN7695_TransAutoNeutralRequest','SPN4255_TransRequestedLaunchGear','SPN2985_TransShiftSelDispModeSw','SPN4246_TransmissionMode5','SPN4247_TransmissionMode6','SPN4248_TransmissionMode7','SPN4249_TransmissionMode8'}},'InputPortsDataType',{{'SS_DOUBLE','SS_DOUBLE','SS_DOUBLE','SS_DOUBLE','SS_DOUBLE','SS_DOUBLE','SS_DOUBLE','SS_DOUBLE','SS_DOUBLE','SS_DOUBLE','SS_DOUBLE','SS_DOUBLE','SS_DOUBLE','SS_DOUBLE','SS_DOUBLE','SS_DOUBLE','SS_DOUBLE','SS_DOUBLE','SS_DOUBLE','SS_DOUBLE','SS_DOUBLE','SS_DOUBLE','SS_DOUBLE','SS_DOUBLE','SS_DOUBLE'}},'OutputPortsWidth',int32([1 1 1 1]),'OutputPortsActive',[1 1 1 1],'OutputPortsName',{{['TX status'],['TX time'],['TX delta time'],['TX delay time']}},'DialogFcn','rtican_message_interface_gui','BlockDisplay',{{'','center'}},'IconTransparency','on','InitLevel',3,'BlockName',struct('Token',{{'TC1_03_05'}}),'SampleTime',{{-1}},'TriggerPort',{{'none'}},'EnablePort',{{'yes'}})  RTIBlockParameters="struct('BoardTypeNo',{{1,'OFF',[]}},'BoardNo',{{1,'ON',[1 16]}},'ChannelNo',{{1,'ON',[1 2]}},'Parameters',{{struct('DataFileSupport',struct('DataFileSelectedMaster',1,'DataFileSelectedLocal',0,'DataFileName',['c:\\users\\gavin.coelho\\repos\\l4 svn\\branches\\gennaro\\project_l4\\src\\projectlibrary\\dbc\\mabx_can1.dbc|c:\\users\\gavin.coelho\\repos\\l4 svn\\branches\\gennaro\\project_l4\\src\\projectlibrary\\dbc\\j1939_famosdbcwithfusion.dbc|'],'DataFileDate',{{{''}}},'SelectedFile',['<no file selected>']),'Options',struct('StatusSelected',1,'TimeSelected',1,'DeltaTimeSelected',1,'DelayTimeSelected',1,'DelayTimeTXCommandSelected',0,'EncodeSetUnusedBitsToOne',0,'EnableMsgLoopback',0,'TriggerPort',struct('Selected',0,'TriggerType',0),'EnablePortSelected',1,'SignalOnPortnameSelected',1,'UserCoding',struct('Selected',0,'InterfaceFile','UserEncodingFile','FcnName','UserEncodeFcn','InportSelected',0,'InportWidth',1,'OutportSelected',0,'OutportWidth',1),'TerminationMsg',struct('Selected',0,'Byte0_7','0'),'InitialMsg',struct('Selected',0,'Byte0_7','0')),'Message',struct('MsgOnBlocknameSelected',1,'MsgName','TC1_03_05','MsgIdFormat',1,'MsgId',201392901,'MsgLength',8,'NumSignals',25,'SampleTime',-1,'StartTime',struct('Selected',0,'Value',0),'AutoRepeatTime',struct('Selected',0,'Value',0.1),'Timeout',struct('Selected',0,'Value',0.1),'DelayTime',struct('Selected',0,'Value',0.1),'Signal',struct('SgnName',{'SPN681_TransGearShiftInhibitReq','SPN682_TransTrqConvLockupDisReq','SPN683_DisengageDrivelineReq','SPN4242_TransRevGearShiftInhibRq','SPN684_RequestedPercClutchSlip','SPN525_TransRequestedGear','SPN685_DisengageDiffLockRqFrAx1','SPN686_DisengageDiffLockRqFrAx2','SPN687_DisengageDiffLockRqRrAx1','SPN688_DisengageDiffLockRqRrAx2','SPN689_DisengageDiffLockRqC','SPN690_DisengageDiffLockRqCF','SPN691_DisengageDiffLockRqCR','SPN5762_TransLoadRedInhibitRq','SPN1852_TransmissionMode1','SPN1853_TransmissionMode2','SPN1854_TransmissionMode3','SPN1855_TransmissionMode4','SPN7695_TransAutoNeutralRequest','SPN4255_TransRequestedLaunchGear','SPN2985_TransShiftSelDispModeSw','SPN4246_TransmissionMode5','SPN4247_TransmissionMode6','SPN4248_TransmissionMode7','SPN4249_TransmissionMode8'},'SgnStartBit',{0,2,4,6,8,16,24,26,28,30,32,34,36,38,40,42,44,46,48,50,54,56,58,60,62},'SgnLength',{2,2,2,2,8,8,2,2,2,2,2,2,2,2,2,2,2,2,2,4,2,2,2,2,2},'SgnType',{0,0,0,0,0,0,0,0,0,0,0,0,0,0,0,0,0,0,0,0,0,0,0,0,0},'ModeValue',{-1,-1,-1,-1,-1,-1,-1,-1,-1,-1,-1,-1,-1,-1,-1,-1,-1,-1,-1,-1,-1,-1,-1,-1,-1},'DataType',{0,0,0,0,0,0,0,0,0,0,0,0,0,0,0,0,0,0,0,0,0,0,0,0,0},'ByteLayout',{0,0,0,0,0,0,0,0,0,0,0,0,0,0,0,0,0,0,0,0,0,0,0,0,0},'Factor',{1,1,1,1,0.4,1,1,1,1,1,1,1,1,1,1,1,1,1,1,1,1,1,1,1,1},'Offset',{0,0,0,0,0,-125,0,0,0,0,0,0,0,0,0,0,0,0,0,0,0,0,0,0,0},'SgnComment',{{['Command signal to inhibit gear shifts.']},{['Command signal to prevent torque converter lockup, which may cause problems in certain circumstances for ASR.']},{''},{['Allows devices external to the normal transmission shift selector system to request the transmission to inhibit shifts into any Reverse gear and force the transmission into Neutral if it is currently in Reverse or attempting to shift to Reverse.']},{['Parameter which represents the percent clutch slip requested by a device.']},{['Gear requested by the operator, ABS, or engine.']},{['Command signal used to disengage the various differential locks, e.g., to allow an undistributed individual wheel control by ABS.  The differential locks are located as defined in Figure SPN564_A.']},{['Command signal used to disengage the various differential locks, e.g., to allow an undistributed individual wheel control by ABS.  The differential locks are located as defined in Figure SPN564_A']},{['Command signal used to disengage the various differential locks, e.g., to allow an undistributed individual wheel control by ABS.  The differential locks are located as defined in Figure SPN564_A']},{['Command signal used to disengage the various differential locks, e.g., to allow an undistributed individual wheel control by ABS.  The differential locks are located as defined in Figure SPN564_A']},{['Command signal used to disengage the various differential locks, e.g., to allow an undistributed individual wheel control by ABS.  The differential locks are located as defined in Figure SPN564_A']},{['Command signal used to disengage the various differential locks, e.g., to allow an undistributed individual wheel control by ABS.  The differential locks are located as defined in Figure SPN564_A.']},{['Command signal used to disengage the various differential locks, e.g., to allow an undistributed individual wheel control by ABS.  The differential locks are located as defined in Figure SPN564_A.']},{['Request signal to the transmission to inhibit activation of load reduction functions.']},{['Indicates whether transmission mode 1 is enabled.  Modes are manufacturer specific and are not necessarily mutually exclusive.  See also SPN 2536.']},{['Indicates whether transmission mode 2 is enabled.  Modes are manufacturer specific and are not necessarily mutually exclusive.  See also SPN 2537.']},{['Indicates whether transmission mode 3 is enabled.  Modes are manufacturer specific and are not necessarily mutually exclusive.  See also SPN 2538.']},{['Indicates whether transmission mode 4 is enabled.  Modes are manufacturer specific and are not necessarily mutually exclusive.  See also SPN 2539.']},{['This parameter conveys a vehicle system desire to override the operator’s current shift selector request (e.g. Drive, Reverse) and shift the transmission into Neutral']},{['Initial gear for the transmission to start out in when the vehicle is launched from a standing stop, as specified by the vehicle operator or vehicle system.']},{['Status of the operator’s switch used to ‘toggle’ through multiple display modes of a shift selector display.']},{['Indicates whether transmission mode 5 is enabled. Modes are manufacturer specific and are not necessarily mutually exclusive. See also SPN 4250.']},{['Indicates whether transmission mode 6 is enabled. Modes are manufacturer specific and are not necessarily mutually exclusive. See also SPN 4251.']},{['Indicates whether transmission mode 7 is enabled. Modes are manufacturer specific and are not necessarily mutually exclusive. See also SPN 4252.']},{['Indicates whether transmission mode 8 is enabled. Modes are manufacturer specific and are not necessarily mutually exclusive. See also SPN 4253.']}},'SgnUnit',{'','','','','%','','','','','','','','','','','','','','','','','','','',''},'Min',{0,0,0,0,0,0,0,0,0,0,0,0,0,0,0,0,0,0,0,0,0,0,0,0,0},'Max',{0,0,0,0,0,0,0,0,0,0,0,0,0,0,0,0,0,0,0,0,0,0,0,0,0},'SLDataType',{'SS_DOUBLE','SS_DOUBLE','SS_DOUBLE','SS_DOUBLE','SS_DOUBLE','SS_DOUBLE','SS_DOUBLE','SS_DOUBLE','SS_DOUBLE','SS_DOUBLE','SS_DOUBLE','SS_DOUBLE','SS_DOUBLE','SS_DOUBLE','SS_DOUBLE','SS_DOUBLE','SS_DOUBLE','SS_DOUBLE','SS_DOUBLE','SS_DOUBLE','SS_DOUBLE','SS_DOUBLE','SS_DOUBLE','SS_DOUBLE','SS_DOUBLE'}),'MsgIdNumFormat',1,'MsgComment',{{['Transmission Control 1']}}),'Version',1.2,'general',struct('isFromLib',0)),'OFF',[]}},'GroupId',{{struct('Group',{{'RTICAN'}},'No',1,'Behavior',{{'NAMECHANGE'}},'BlockType',{{'SINK'}},'NameChangeFlag',0),'OFF',[]}},'SFcnRTICANMessage',{{struct('MsgType','TX','SFcnPortType','Scalar','MsgName','TC1_03_05','MsgIdFormat','XTD','MsgId',201392901,'MsgLength',8,'NumSignals',25,'SampleTime',-1,'StartTime',struct('Selected','no','Value',0),'AutoRepeatTime',struct('Selected','no','Value',0.1),'Timeout',struct('Selected','no','Value',0.1),'Signal',struct('SgnName',{'SPN681_TransGearShiftInhibitReq','SPN682_TransTrqConvLockupDisReq','SPN683_DisengageDrivelineReq','SPN4242_TransRevGearShiftInhibRq','SPN684_RequestedPercClutchSlip','SPN525_TransRequestedGear','SPN685_DisengageDiffLockRqFrAx1','SPN686_DisengageDiffLockRqFrAx2','SPN687_DisengageDiffLockRqRrAx1','SPN688_DisengageDiffLockRqRrAx2','SPN689_DisengageDiffLockRqC','SPN690_DisengageDiffLockRqCF','SPN691_DisengageDiffLockRqCR','SPN5762_TransLoadRedInhibitRq','SPN1852_TransmissionMode1','SPN1853_TransmissionMode2','SPN1854_TransmissionMode3','SPN1855_TransmissionMode4','SPN7695_TransAutoNeutralRequest','SPN4255_TransRequestedLaunchGear','SPN2985_TransShiftSelDispModeSw','SPN4246_TransmissionMode5','SPN4247_TransmissionMode6','SPN4248_TransmissionMode7','SPN4249_TransmissionMode8'},'SgnStartBit',{0,2,4,6,8,16,24,26,28,30,32,34,36,38,40,42,44,46,48,50,54,56,58,60,62},'SgnLength',{2,2,2,2,8,8,2,2,2,2,2,2,2,2,2,2,2,2,2,4,2,2,2,2,2},'SgnType',{'standard','standard','standard','standard','standard','standard','standard','standard','standard','standard','standard','standard','standard','standard','standard','standard','standard','standard','standard','standard','standard','standard','standard','standard','standard'},'ModeValue',{-1,-1,-1,-1,-1,-1,-1,-1,-1,-1,-1,-1,-1,-1,-1,-1,-1,-1,-1,-1,-1,-1,-1,-1,-1},'DataType',{['unsigned int'],['unsigned int'],['unsigned int'],['unsigned int'],['unsigned int'],['unsigned int'],['unsigned int'],['unsigned int'],['unsigned int'],['unsigned int'],['unsigned int'],['unsigned int'],['unsigned int'],['unsigned int'],['unsigned int'],['unsigned int'],['unsigned int'],['unsigned int'],['unsigned int'],['unsigned int'],['unsigned int'],['unsigned int'],['unsigned int'],['unsigned int'],['unsigned int']},'ByteLayout',{['little endian'],['little endian'],['little endian'],['little endian'],['little endian'],['little endian'],['little endian'],['little endian'],['little endian'],['little endian'],['little endian'],['little endian'],['little endian'],['little endian'],['little endian'],['little endian'],['little endian'],['little endian'],['little endian'],['little endian'],['little endian'],['little endian'],['little endian'],['little endian'],['little endian']},'Factor',{1,1,1,1,0.4,1,1,1,1,1,1,1,1,1,1,1,1,1,1,1,1,1,1,1,1},'Offset',{0,0,0,0,0,-125,0,0,0,0,0,0,0,0,0,0,0,0,0,0,0,0,0,0,0},'SLDataType',{'SS_DOUBLE','SS_DOUBLE','SS_DOUBLE','SS_DOUBLE','SS_DOUBLE','SS_DOUBLE','SS_DOUBLE','SS_DOUBLE','SS_DOUBLE','SS_DOUBLE','SS_DOUBLE','SS_DOUBLE','SS_DOUBLE','SS_DOUBLE','SS_DOUBLE','SS_DOUBLE','SS_DOUBLE','SS_DOUBLE','SS_DOUBLE','SS_DOUBLE','SS_DOUBLE','SS_DOUBLE','SS_DOUBLE','SS_DOUBLE','SS_DOUBLE'}),'StatusSelected','yes','TimeSelected','yes','DeltaTimeSelected','yes','DelayTimeSelected','yes','DelayTimeTXCommandSelected','no','EncodeSetUnusedBitsToOne','no','EnableMsgLoopback','no','TriggerPort',struct('Selected','no','TriggerType',0),'EnablePortSelected','yes','UserCoding',struct('Selected','no','InterfaceFile','UserEncodingFile','FcnName','UserEncodeFcn','InportSelected','no','InportWidth',1,'OutportSelected','no','OutportWidth',1),'TerminationMsg',struct('Selected','no','Byte0','0x00','Byte1','0x00','Byte2','0x00','Byte3','0x00','Byte4','0x00','Byte5','0x00','Byte6','0x00','Byte7','0x00'),'InitialMsg',struct('Selected','no','Byte0','0x00','Byte1','0x00','Byte2','0x00','Byte3','0x00','Byte4','0x00','Byte5','0x00','Byte6','0x00','Byte7','0x00'),'BoardType','DS1','BoardNo',1,'ControllerNo',1),'OFF',[]}},'TLCFileName',{{'rtican_tx_message','OFF',[]}})"  RTISFcnParameters=struct('SFcnRTICANMessage','struct','TLCFileName','char')  RTIBlockParaDefault=struct('BoardTypeNo',4302,'BoardNo',1,'ChannelNo',1,'Parameters',struct('DataFileSupport',struct('DataFileSelectedMaster',0,'DataFileSelectedLocal',0,'DataFileName','','DataFileDate','','SelectedFile',['<no file selected>']),'Options',struct('StatusSelected',1,'TimeSelected',1,'DeltaTimeSelected',1,'DelayTimeSelected',1,'DelayTimeTXCommandSelected',0,'EncodeSetUnusedBitsToOne',0,'EnableMsgLoopback',0,'TriggerPort',struct('Selected',0,'TriggerType','rising'),'EnablePortSelected',0,'SignalOnPortnameSelected',1,'UserCoding',struct('Selected',0,'InterfaceFile','UserEncodingFile','FcnName','UserEncodeFcn','InportSelected',0,'InportWidth',1,'OutportSelected',0,'OutportWidth',1),'TerminationMsg',struct('Selected',0,'Byte0_7','0'),'InitialMsg',struct('Selected',0,'Byte0_7','0')),'Message',struct('MsgOnBlocknameSelected',0,'MsgName',['TX Message'],'MsgIdFormat',0,'MsgId',100,'MsgLength',8,'NumSignals',1,'SampleTime',-1,'StartTime',struct('Selected',0,'Value',0),'AutoRepeatTime',struct('Selected',0,'Value',0.1),'Timeout',struct('Selected',0,'Value',0.1),'DelayTime',struct('Selected',0,'Value',0.1),'Signal',struct('SgnName',['TX signal'],'SgnStartBit',0,'SgnLength',8,'SgnType',0,'ModeValue',-1,'DataType',0,'SLDataType','SS_DOUBLE','ByteLayout',0,'Factor',1,'Offset',0,'Min',0,'Max',255,'SgnComment',{{}},'SgnUnit',''),'MsgIdNumFormat',0,'MsgComment',{{''}}),'Version',1.2,'general',struct('isFromLib',1)),'GroupId',struct('Group',{{'RTICAN'}},'No',1,'Behavior',{{'NAMECHANGE'}},'BlockType',{{'SINK'}},'NameChangeFlag',0),'SFcnRTICANMessage',struct('MsgType','TX','MsgName',['TX Message'],'MsgIdFormat','STD','MsgId',100,'MsgLength',2,'NumSignals',1,'SampleTime',-1,'StartTime',struct('Selected','no','Value',0),'AutoRepeatTime',struct('Selected','no','Value',0.1),'Timeout',struct('Selected','no','Value',0.1),'DelayTime',struct('Selected','no','Value',0.1),'Signal',struct('SgnName',['TX signal'],'SgnStartBit',0,'SgnLength',8,'SgnType','standard','ModeValue',-1,'DataType',['unsigned int'],'ByteLayout',['little endian'],'SLDataType','SS_DOUBLE','Factor',1,'Offset',0),'StatusSelected','yes','TimeSelected','yes','DeltaTimeSelected','yes','DelayTimeSelected','yes','EnablePortSelected','no','EnableMsgLoopback','no','DelayTimeTXCommandSelected','no','EncodeSetUnusedBitsToOne','no','UserCoding',struct('Selected','no','InterfaceFile','UserDecodingFile','FcnName','UserDecodeFcn','InportSelected','no','InportWidth',1,'OutportSelected','no','OutportWidth',1),'TerminationMsg',struct('Selected','no','Byte0','0x00','Byte1','0x00','Byte2','0x00','Byte3','0x00','Byte4','0x00','Byte5','0x00','Byte6','0x00','Byte7','0x00'),'InitialMsg',struct('Selected','no','Byte0','0x00','Byte1','0x00','Byte2','0x00','Byte3','0x00','Byte4','0x00','Byte5','0x00','Byte6','0x00','Byte7','0x00'),'TriggerPort',struct('Selected','no','TriggerType','rising'),'BoardType','DS4302','BoardNo',1,'ControllerNo',1,'SFcnPortType','Scalar'),'TLCFileName','rtican_tx_message')
      settings: AttributesFormatString=Group Id: RTICAN1\n  SourceProductName=dSPACE RTI CAN Blockset
  Terminator{,1..4} (5 alike) : Terminator
  wires:
  In1/1 -> Bus Selector/1
  TC1_03_05/4 -> Terminator3/1
  TC1_03_05/3 -> Terminator2/1
  TC1_03_05/2 -> Terminator1/1
  TC1_03_05/1 -> Terminator/1
  Bus Selector/25 -> TC1_03_05/25  "<SPN4249_TransmissionMode8>"
  Bus Selector/24 -> TC1_03_05/24  "<SPN4248_TransmissionMode7>"
  Bus Selector/23 -> TC1_03_05/23  "<SPN4247_TransmissionMode6>"
  Bus Selector/22 -> TC1_03_05/22  "<SPN4246_TransmissionMode5>"
  Bus Selector/21 -> TC1_03_05/21  "<SPN2985_TransShiftSelDispModeSw>"
  Bus Selector/20 -> TC1_03_05/20  "<SPN4255_TransRequestedLaunchGear>"
  Bus Selector/19 -> TC1_03_05/19  "<SPN7695_TransAutoNeutralRequest>"
  Bus Selector/18 -> TC1_03_05/18  "<SPN1855_TransmissionMode4>"
  Bus Selector/17 -> TC1_03_05/17  "<SPN1854_TransmissionMode3>"
  Bus Selector/16 -> TC1_03_05/16  "<SPN1853_TransmissionMode2>"
  Bus Selector/15 -> TC1_03_05/15  "<SPN1852_TransmissionMode1>"
  Bus Selector/14 -> TC1_03_05/14  "<SPN5762_TransLoadRedInhibitRq>"
  Bus Selector/13 -> TC1_03_05/13  "<SPN691_DisengageDiffLockRqCR>"
  Bus Selector/12 -> TC1_03_05/12  "<SPN690_DisengageDiffLockRqCF>"
  Bus Selector/11 -> TC1_03_05/11  "<SPN689_DisengageDiffLockRqC>"
  Bus Selector/10 -> TC1_03_05/10  "<SPN688_DisengageDiffLockRqRrAx2>"
  Bus Selector/9 -> TC1_03_05/9  "<SPN687_DisengageDiffLockRqRrAx1>"
  Bus Selector/8 -> TC1_03_05/8  "<SPN686_DisengageDiffLockRqFrAx2>"
  Bus Selector/7 -> TC1_03_05/7  "<SPN685_DisengageDiffLockRqFrAx1>"
  Bus Selector/6 -> TC1_03_05/6  "<SPN525_TransRequestedGear>"
  Bus Selector/5 -> TC1_03_05/5  "<SPN684_RequestedPercClutchSlip>"
  Bus Selector/4 -> TC1_03_05/4  "<SPN4242_TransRevGearShiftInhibRq>"
  Bus Selector/3 -> TC1_03_05/3  "<SPN683_DisengageDrivelineReq>"
  Bus Selector/2 -> TC1_03_05/2  "<SPN682_TransTrqConvLockupDisReq>"
  Bus Selector/1 -> TC1_03_05/1  "<SPN681_TransGearShiftInhibitReq>"
  Bus Selector/26 -> Terminator4/1  "<RX_status>"
  CANT_TC1_03_05_APV/1 -> TC1_03_05/Enable

== system SUB_ECU_L4_MABX_HW_Interface_PIC_KW/CAN_Out_PIC_KW/CAN_TX_BAM/CM ==
  Byte1 : Constant  Value=hex2dec('20')  OutDataTypeStr=uint8
  Byte2 : Constant  Value=hex2dec('D')  OutDataTypeStr=uint8
  Byte3 : Constant  Value=hex2dec('0')  OutDataTypeStr=uint8
  Byte4 : Constant  Value=hex2dec('2')  OutDataTypeStr=uint8
  Byte5 : Constant  Value=hex2dec('FF')  OutDataTypeStr=uint8
  Byte6 : Constant  Value=hex2dec('EB')  OutDataTypeStr=uint8
  Byte7 : Constant  Value=hex2dec('FE')  OutDataTypeStr=uint8
  Byte8 : Constant  Value=hex2dec('0')  OutDataTypeStr=uint8
  Vector Concatenate : Concatenate  NumInputs=8
  Out1 : Outport
  wires:
  Byte2/1 -> Vector Concatenate/2
  Byte5/1 -> Vector Concatenate/5
  Byte3/1 -> Vector Concatenate/3
  Byte6/1 -> Vector Concatenate/6
  Vector Concatenate/1 -> Out1/1
  Byte4/1 -> Vector Concatenate/4
  Byte1/1 -> Vector Concatenate/1
  Byte8/1 -> Vector Concatenate/8
  Byte7/1 -> Vector Concatenate/7

== system SUB_ECU_L4_MABX_HW_Interface_PIC_KW/CAN_Out_PIC_KW/CAN_TX_BAM/DataFrame1 ==
  Byte1 : Constant  Value=hex2dec('1')  OutDataTypeStr=uint8
  Byte2 : Constant  Value=uint8('P')  OutDataTypeStr=uint8
  Byte3 : Constant  Value=uint8('C')  OutDataTypeStr=uint8
  Byte4 : Constant  Value=uint8('A')  OutDataTypeStr=uint8
  Byte5 : Constant  Value=uint8('R')  OutDataTypeStr=uint8
  Byte6 : Constant  Value=uint8('*')  OutDataTypeStr=uint8
  Byte7 : Constant  Value=uint8('R')  OutDataTypeStr=uint8
  Byte8 : Constant  Value=uint8('N')  OutDataTypeStr=uint8
  Vector Concatenate : Concatenate  NumInputs=8
  Out1 : Outport
  wires:
  Byte7/1 -> Vector Concatenate/7
  Byte8/1 -> Vector Concatenate/8
  Byte1/1 -> Vector Concatenate/1
  Byte4/1 -> Vector Concatenate/4
  Vector Concatenate/1 -> Out1/1
  Byte6/1 -> Vector Concatenate/6
  Byte3/1 -> Vector Concatenate/3
  Byte5/1 -> Vector Concatenate/5
  Byte2/1 -> Vector Concatenate/2

== system SUB_ECU_L4_MABX_HW_Interface_PIC_KW/CAN_Out_PIC_KW/CAN_TX_BAM/DataFrame2 ==
  Byte1 : Constant  Value=hex2dec('2')  OutDataTypeStr=uint8
  Byte2 : Constant  Value=uint8('D')  OutDataTypeStr=uint8
  Byte3 : Constant  Value=uint8('M')  OutDataTypeStr=uint8
  Byte4 : Constant  Value=uint8('L')  OutDataTypeStr=uint8
  Byte5 : Constant  Value=uint8('*')  OutDataTypeStr=uint8
  Byte6 : Constant  Value=uint8('*')  OutDataTypeStr=uint8
  Byte7 : Constant  Value=uint8(255)  OutDataTypeStr=uint8
  Byte8 : Constant  Value=uint8(255)  OutDataTypeStr=uint8
  Vector Concatenate : Concatenate  NumInputs=8
  Out1 : Outport
  wires:
  Byte2/1 -> Vector Concatenate/2
  Byte5/1 -> Vector Concatenate/5
  Byte3/1 -> Vector Concatenate/3
  Byte6/1 -> Vector Concatenate/6
  Vector Concatenate/1 -> Out1/1
  Byte4/1 -> Vector Concatenate/4
  Byte1/1 -> Vector Concatenate/1
  Byte8/1 -> Vector Concatenate/8
  Byte7/1 -> Vector Concatenate/7
